simulink model "hardware_IOTest_CBF"  (R2024a)
settings: Solver=FixedStepAuto  StartTime=0.0  StopTime=inf  FixedStep=1/30  RelTol=1e-3  EnableMultiTasking=on
undefined symbols (not defined in the file): qc_get_step_size
libraries: quarc_library x4
settings Model: SimulationMode=external  Creator=kfullerton  LastModifiedBy=Dell
settings SolverCC: PositivePriorityOrder=on
settings OptimizationCC: ReuseModelBlockBuffer=off
settings HardwareCC: ProdBitPerLong=64  ProdLargestAtomicInteger=LongLong  ProdLargestAtomicFloat=Double  ProdLongLongMode=on  ProdHWDeviceType=ARM Compatible->ARM 64-bit (LP64)
settings ModelReferenceCC: EnableRefExpFcnMdlSchedulingChecks=on
settings RTWCC: Description=QUARC Linux Raspberry Pi Arm64 Target (QBot Platform) Using Toolchain  SystemTargetFile=quarc_linux_pi_arm64.tlc  Toolchain=QUARC linux_pi_arm64 | gmake (64-bit Windows)  BuildConfiguration=Faster Runs  GPUComputeCapability=3.5
settings STFCustomTargetCC: ConcurrentExecutionCompliant=on  SystemTargetFile=quarc_linux_pi_arm64.tlc
settings GRTTargetCC: ParMdlRefBuildCompliant=off  CompOptLevelCompliant=off  CombineOutputUpdateFcns=off  MatFileLogging=off  CPPClassGenCompliant=off  GRTInterface=on  ExtMode=on  ExtModeMexFile=quarc_comm  ExtModeMexArgs='-w -d /tmp -uri %u','tcpip://192.168.2.12:17002'

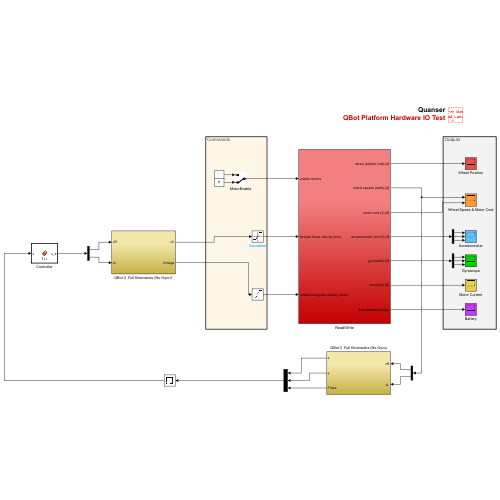
[thumbnail: Simulink's stored preview of the top-level diagram]
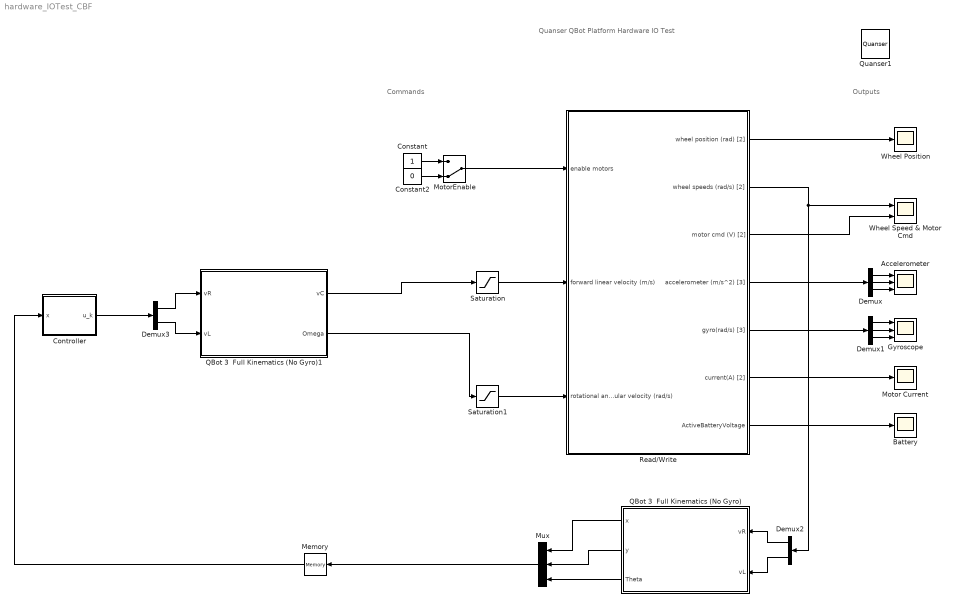
== system hardware_IOTest_CBF ==
  note: Outputs
  note: Commands
  note: Quanser
      | QBot Platform Hardware IO Test
  Accelerometer : Scope  NumInputPorts=3
  Battery : Scope
  Constant : Constant
  Constant2 : Constant  Value=0
  Controller : MATLAB Function  TreatAsAtomicUnit=on
  Demux : Demux  Outputs=3
  Demux1 : Demux  Outputs=3
  Demux2 : Demux  Outputs=2
  Demux3 : Demux  Outputs=2
  Gyroscope : Scope  NumInputPorts=3
  Memory : Memory  InitialCondition=[5,5,9]
  Motor Current : Scope
  MotorEnable : ManualSwitch  InitFcn=set_param(gcb,'sw','0')  CurrentSetting=0
  Mux : Mux  Inputs=3
  QBot 3  Full Kinematics (No Gyro) : Subsystem
  QBot 3  Full Kinematics (No Gyro)1 : Subsystem
  Quanser1 : quarc_library/Logos/Quanser
  Read/Write : Subsystem
  Saturation : Saturate  UpperLimit=0.7  LowerLimit=-0.7
  Saturation1 : Saturate  UpperLimit=3.564  LowerLimit=-3.564
  Wheel Position : Scope
  Wheel Speed & Motor Cmd : Scope  NumInputPorts=2
  wires:
  MotorEnable/1 -> Read/Write/1(enable motors)
  Constant/1 -> MotorEnable/1
  QBot 3  Full Kinematics (No Gyro)1/2(Omega) -> Saturation1/1
  Read/Write/2(wheel speeds (rad/s) [2]) -> Demux2/1, Wheel Speed & Motor Cmd/1
  Read/Write/3(motor cmd (V) [2]) -> Wheel Speed & Motor Cmd/2
  Read/Write/1(wheel position (rad) [2]) -> Wheel Position/1
  Read/Write/4(accelerometer (m/s^2) [3]) -> Demux/1
  Demux/1 -> Accelerometer/1
  Demux/2 -> Accelerometer/2
  Demux/3 -> Accelerometer/3
  Demux1/1 -> Gyroscope/1
  Read/Write/5(gyro(rad/s) [3]) -> Demux1/1
  Demux1/3 -> Gyroscope/3
  Demux1/2 -> Gyroscope/2
  Read/Write/6(current(A) [2]) -> Motor Current/1
  Read/Write/7(ActiveBatteryVoltage) -> Battery/1
  Constant2/1 -> MotorEnable/2
  Saturation/1 -> Read/Write/2(forward linear velocity (m/s))
  Saturation1/1 -> Read/Write/3(rotational angular velocity (rad/s))
  Demux2/1 -> QBot 3  Full Kinematics (No Gyro)/1(vR)
  Demux2/2 -> QBot 3  Full Kinematics (No Gyro)/2(vL)
  QBot 3  Full Kinematics (No Gyro)/1(x) -> Mux/1
  QBot 3  Full Kinematics (No Gyro)/2(y) -> Mux/2
  QBot 3  Full Kinematics (No Gyro)/3(Theta) -> Mux/3
  Mux/1 -> Memory/1
  Memory/1 -> Controller/1(x)
  Controller/1(u_k) -> Demux3/1
  Demux3/1 -> QBot 3  Full Kinematics (No Gyro)1/1(vR)
  Demux3/2 -> QBot 3  Full Kinematics (No Gyro)1/2(vL)
  QBot 3  Full Kinematics (No Gyro)1/1(vC) -> Saturation/1

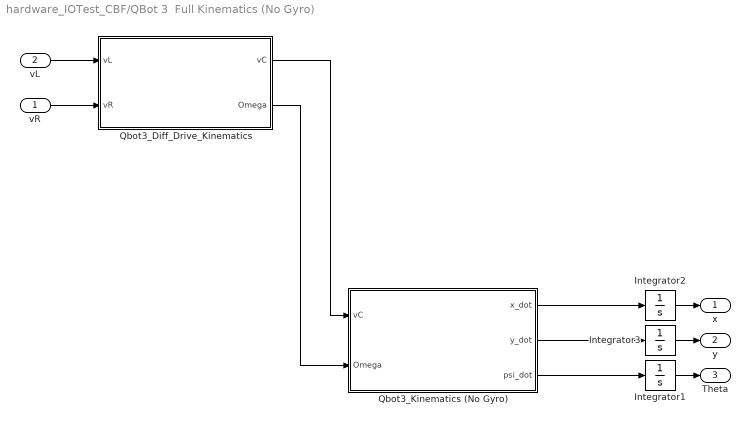
== system hardware_IOTest_CBF/QBot 3  Full Kinematics (No Gyro) ==
  vR : Inport
  vL : Inport  Port=2
  Integrator1 : Integrator
  Integrator2 : Integrator
  Integrator3 : Integrator
  Qbot3_Diff_Drive_Kinematics : Subsystem
  Qbot3_Kinematics (No Gyro) : Subsystem
  x : Outport
  y : Outport  Port=2
  Theta : Outport  Port=3
  wires:
  Integrator1/1 -> Theta/1
  Integrator2/1 -> x/1
  Integrator3/1 -> y/1
  Qbot3_Kinematics (No Gyro)/3(psi_dot) -> Integrator1/1
  vR/1 -> Qbot3_Diff_Drive_Kinematics/2(vR)
  Qbot3_Diff_Drive_Kinematics/1(vC) -> Qbot3_Kinematics (No Gyro)/1(vC)
  Qbot3_Diff_Drive_Kinematics/2(Omega) -> Qbot3_Kinematics (No Gyro)/2(Omega)
  vL/1 -> Qbot3_Diff_Drive_Kinematics/1(vL)
  Qbot3_Kinematics (No Gyro)/1(x_dot) -> Integrator2/1
  Qbot3_Kinematics (No Gyro)/2(y_dot) -> Integrator3/1

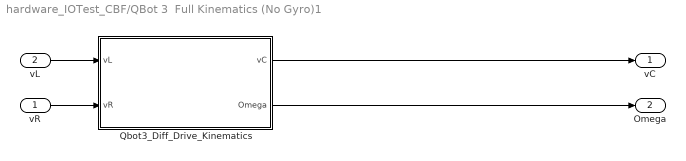
== system hardware_IOTest_CBF/QBot 3  Full Kinematics (No Gyro)1 ==
  vR : Inport
  vL : Inport  Port=2
  Qbot3_Diff_Drive_Kinematics : Subsystem
  vC : Outport
  Omega : Outport  Port=2
  wires:
  vL/1 -> Qbot3_Diff_Drive_Kinematics/1(vL)
  Qbot3_Diff_Drive_Kinematics/2(Omega) -> Omega/1
  Qbot3_Diff_Drive_Kinematics/1(vC) -> vC/1
  vR/1 -> Qbot3_Diff_Drive_Kinematics/2(vR)

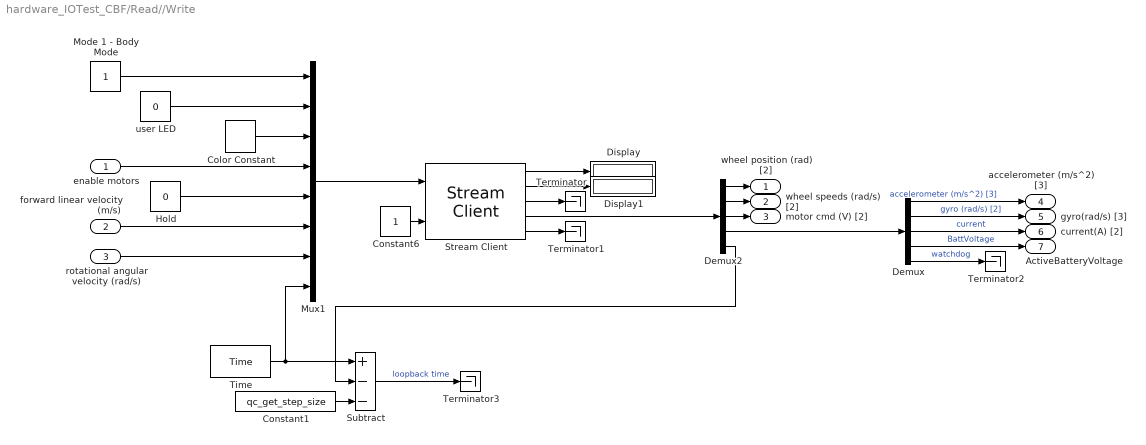
== system hardware_IOTest_CBF/Read//Write ==
  enable motors : Inport
  forward linear velocity (m/s) : Inport  Port=2
  rotational angular velocity (rad/s) : Inport  Port=3
  Color Constant : quarc_library/Sources/Signals/Color Constant  color=[0 1 1]
  Constant1 : Constant  Value=qc_get_step_size
  Constant6 : Constant
  Demux : Demux  Outputs=[3 3 2 1 1]
  Demux2 : Demux  Outputs=[2 2 2 10 1]
  Display : Display
  Display1 : Display
  Hold : Constant  Value=0
  Mode 1 - Body Mode : Constant
  Mux1 : Mux  Inputs=8
  Stream Client : quarc_library/Communications/Basic/Stream Client  uri_source=Specify via dialog (do not evaluate)  uri=tcpip://localhost:18888  send_buffer_size=1460  receive_buffer_size=1460  byte_order=little endian (Intel - LSB first)  optimization=Minimum latency  send_options=Send most recent data  receive_options=Receive most recent data  default_value=zeros(17,1)  sample_time=qc_get_step_size  active=off  implementation=Use blocking I/O in a separate thread  send_fifo_size=1000  receive_fifo_size=1000  send_priority=0  receive_priority=0  send_dimensions=off  receive_dimensions=off  max_dimensions=-1  data_type=Inherited via back propagation  type_expr=BusObject
      settings: AttributesFormatString="\"tcpip://localhost:18888\""
  Subtract : Sum  Inputs=+--
  Terminator{,1..3} (4 alike) : Terminator
  Time : quarc_library/Sources/Time/Time  time_source=Wall clock  sample_time=qc_get_step_size
  user LED : Constant  Value=0
  wheel position (rad) [2] : Outport
  wheel speeds (rad/s) [2] : Outport  Port=2
  motor cmd (V) [2] : Outport  Port=3
  accelerometer (m/s^2) [3] : Outport  Port=4
  gyro(rad/s) [3] : Outport  Port=5
  current(A) [2] : Outport  Port=6
  ActiveBatteryVoltage : Outport  Port=7
  wires:
  Stream Client/5 -> Terminator1/1
  Mode 1 - Body Mode/1 -> Mux1/1
  user LED/1 -> Mux1/2
  enable motors/1 -> Mux1/4
  Demux2/4 -> Demux/1
  Mux1/1 -> Stream Client/1
  Stream Client/2 -> Display1/1
  Stream Client/4 -> Demux2/1
  Stream Client/1 -> Display/1
  forward linear velocity (m/s)/1 -> Mux1/6
  Color Constant/1 -> Mux1/3
  Time/1 -> Mux1/8, Subtract/1
  Constant6/1 -> Stream Client/2
  Subtract/1 -> Terminator3/1  "loopback time"
  Stream Client/3 -> Terminator/1
  Constant1/1 -> Subtract/3
  Demux2/5 -> Subtract/2
  Demux2/3 -> motor cmd (V) [2]/1
  Demux2/1 -> wheel position (rad) [2]/1
  Demux2/2 -> wheel speeds (rad/s) [2]/1
  rotational angular velocity (rad/s)/1 -> Mux1/7
  Demux/1 -> accelerometer (m/s^2) [3]/1  "accelerometer (m/s^2) [3]"
  Demux/2 -> gyro(rad/s) [3]/1  "gyro (rad/s) [2]"
  Demux/4 -> ActiveBatteryVoltage/1  "BattVoltage"
  Demux/3 -> current(A) [2]/1  "current"
  Hold/1 -> Mux1/5
  Demux/5 -> Terminator2/1  "watchdog"

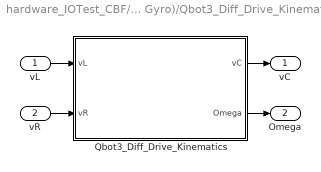
== system hardware_IOTest_CBF/QBot 3  Full Kinematics (No Gyro)/Qbot3_Diff_Drive_Kinematics ==
  vL : Inport
  vR : Inport  Port=2
  Qbot3_Diff_Drive_Kinematics : MATLAB Function  TreatAsAtomicUnit=on
  vC : Outport
  Omega : Outport  Port=2
  wires:
  Qbot3_Diff_Drive_Kinematics/2(Omega) -> Omega/1
  vR/1 -> Qbot3_Diff_Drive_Kinematics/2(vR)
  Qbot3_Diff_Drive_Kinematics/1(vC) -> vC/1
  vL/1 -> Qbot3_Diff_Drive_Kinematics/1(vL)

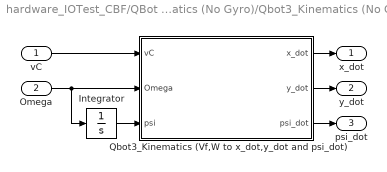
== system hardware_IOTest_CBF/QBot 3  Full Kinematics (No Gyro)/Qbot3_Kinematics (No Gyro) ==
  vC : Inport
  Omega : Inport  Port=2
  Integrator : Integrator
  Qbot3_Kinematics (Vf,W to x_dot,y_dot and psi_dot) : MATLAB Function  TreatAsAtomicUnit=on
  x_dot : Outport
  y_dot : Outport  Port=2
  psi_dot : Outport  Port=3
  wires:
  Omega/1 -> Qbot3_Kinematics (Vf,W to x_dot,y_dot and psi_dot)/2(Omega), Integrator/1
  Qbot3_Kinematics (Vf,W to x_dot,y_dot and psi_dot)/2(y_dot) -> y_dot/1
  Qbot3_Kinematics (Vf,W to x_dot,y_dot and psi_dot)/3(psi_dot) -> psi_dot/1
  vC/1 -> Qbot3_Kinematics (Vf,W to x_dot,y_dot and psi_dot)/1(vC)
  Qbot3_Kinematics (Vf,W to x_dot,y_dot and psi_dot)/1(x_dot) -> x_dot/1
  Integrator/1 -> Qbot3_Kinematics (Vf,W to x_dot,y_dot and psi_dot)/3(psi)

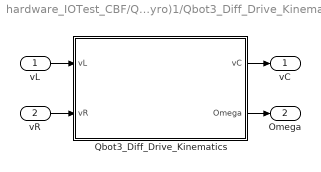
== system hardware_IOTest_CBF/QBot 3  Full Kinematics (No Gyro)1/Qbot3_Diff_Drive_Kinematics ==
  vL : Inport
  vR : Inport  Port=2
  Qbot3_Diff_Drive_Kinematics : MATLAB Function  TreatAsAtomicUnit=on
  vC : Outport
  Omega : Outport  Port=2
  wires:
  vL/1 -> Qbot3_Diff_Drive_Kinematics/1(vL)
  Qbot3_Diff_Drive_Kinematics/1(vC) -> vC/1
  vR/1 -> Qbot3_Diff_Drive_Kinematics/2(vR)
  Qbot3_Diff_Drive_Kinematics/2(Omega) -> Omega/1

== matlab function hardware_IOTest_CBF/QBot 3  Full Kinematics (No Gyro)/Qbot3_Diff_Drive_Kinematics/Qbot3_Diff_Drive_Kinematics ==
  data: vL input; vC output; vR input; Omega output
function [vC,Omega] = fcn(vL,vR)

% wheelbase
d= 0.235;

% calculate forward and turning velocities
vC=0.5*(vL+vR);
Omega=(1/d)*(vR-vL);

== matlab function hardware_IOTest_CBF/Controller ==
  data: x input; u_k output
function u_k = fcn(x)
    coder.extrinsic('opt_problem');
    H = [1,0,0];
    F = -1.5 ;
    u_k=zeros(1,2);
    gaama = 0.5; %0.5
    c = 0.2; %0.2
    d=0.4;
    dist=0.278; % distance between wheels;
    P0 = eye(3);
    P = eye(3);

    theta=x(3);
    A=eye(3);
    D=0.1.*[0.5*cos(theta), 0.5*cos(theta); 0.5*sin(theta), 0.5*sin(theta);1/dist,-1/dist];
    
    q1 = [2 * x' * A * P * D, -1]';
    q2 = [-H * D, 0]';
    r1 = x' * (A' * P * A - P + c * eye(size(A))) * x;
    r2 = -H * (A + (1 - gaama) * eye(size(A))) * x - (2 - gaama) * F;

    P1=zeros(3,3);
    P1(1:2,1:2) = D' * P * D;
    P2 = 0;

    Uk=opt_problem(P0,P1,P2,q1,q2,r1,r2,d);
    u_k=Uk(1:2);
    d=Uk(3);
end

== matlab function hardware_IOTest_CBF/QBot 3  Full Kinematics (No Gyro)1/Qbot3_Diff_Drive_Kinematics/Qbot3_Diff_Drive_Kinematics ==
  data: vL input; vC output; vR input; Omega output
function [vC,Omega] = fcn(vL,vR)

% wheelbase
d= 0.235;

% calculate forward and turning velocities
vC=0.5*(vL+vR);
Omega=(1/d)*(vR-vL);

== matlab function hardware_IOTest_CBF/QBot 3  Full Kinematics (No Gyro)/Qbot3_Kinematics (No Gyro)/Qbot3_Kinematics (Vf,W to x_dot,y_dot and psi_dot) ==
  data: vC input; x_dot output; Omega input; y_dot output; psi input; psi_dot output
function [x_dot,y_dot,psi_dot] = fcn(vC,Omega,psi)

% calculate cartesian velocities
x_dot=cos(psi)*vC;
y_dot=sin(psi)*vC;
psi_dot= Omega;
